simulink model "VOOR"  (R2020a)
settings: Solver=FixedStepAuto  StartTime=0.0  StopTime=16  FixedStep=1e-3  RelTol=1e-3  EnableMultiTasking=on
settings Model: ExtModeTrigDuration=5  Creator=theodor  LastModifiedBy=theodor
settings OptimizationCC: EnhancedBackFolding=on  PassReuseOutputArgsAs=Individual arguments  ZeroExternalMemoryAtStartup=off  ZeroInternalMemoryAtStartup=off  MaxStackSize=64  OptimizeBlockOrder=speed  DifferentSizesBufferReuse=on  OptimizationCustomize=off  EfficientTunableParamExpr=on
settings DebuggingCC: ParameterTunabilityLossMsg=error
settings HardwareCC: ProdBitPerPointer=32  ProdBitPerSizeT=32  ProdBitPerPtrDiffT=32  ProdLargestAtomicInteger=Long  ProdLargestAtomicFloat=Double  ProdWordSize=32  ProdHWDeviceType=ARM Compatible->ARM Cortex
settings SFSimCC: MATLABDynamicMemAlloc=off
settings RTWCC: SystemTargetFile=ert.tlc  HardwareBoard=NXP FRDM-K64F  TemplateMakefile=ert_default_tmf  Toolchain=GNU Tools for ARM Embedded Processors
settings CodeAppCC: ForceParamTrailComments=on  IgnoreCustomStorageClasses=off  OperatorAnnotations=on  SimulinkDataObjDesc=on  SFDataObjDesc=on  InsertBlockDesc=on

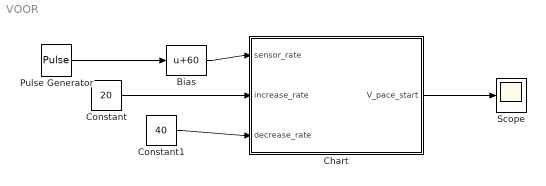
== system VOOR ==
  Bias : Bias  Bias=60
  Chart : Stateflow chart  TreatAsAtomicUnit=on
  Constant : Constant  Value=20
  Constant1 : Constant  Value=40
  Pulse Generator : DiscretePulseGenerator  PulseType=Time based  Amplitude=60  Period=16  PulseWidth=50
  Scope : Scope
  wires:
  Constant/1 -> Chart/2(increase_rate)
  Constant1/1 -> Chart/3(decrease_rate)
  Chart/1(V_pace_start) -> Scope/1
  Pulse Generator/1 -> Bias/1
  Bias/1 -> Chart/1(sensor_rate)

== stateflow chart VOOR/Chart ==
  state INITIAL
    entry:
    current_LRL = sensor_rate;
  state UPDATE_RATE
    on after(1,msec):
    V_pace_start = false;
    exit:
    t = elapsed(sec)
  state PACE
    entry:
    V_pace_start = true;
  (default) -> INITIAL
  INITIAL -> PACE
  (junction 35) -> (junction 37)
  (junction 37) -> (junction 32)
  (junction 13) -> (junction 35) [order 1] : [current_LRL + increase_rate*t > sensor_rate]{current_LRL = sensor_rate}
  (junction 13) -> (junction 32) [order 2] : {current_LRL = current_LRL + increase_rate*t}
  (junction 32) -> UPDATE_RATE
  (junction 42) -> (junction 13) [order 2] : [sensor_rate > current_LRL]
  PACE -> (junction 42)
  (junction 42) -> (junction 14) [order 1] : [sensor_rate <= current_LRL]
  UPDATE_RATE -> PACE : after(60/current_LRL,sec)
  (junction 24) -> UPDATE_RATE
  (junction 14) -> (junction 24) [order 2] : {current_LRL = current_LRL - decrease_rate * t}
  (junction 29) -> (junction 24)
  (junction 14) -> (junction 26) [order 1] : [current_LRL - decrease_rate * t  < sensor_rate ]{current_LRL = sensor_rate}
  (junction 26) -> (junction 29)
  data: V_pace_start output; sensor_rate input; increase_rate input; decrease_rate input; current_LRL local; t local =0
